simulink model "der"  (R2024b)
settings: Solver=VariableStepAuto  StartTime=0.0  StopTime=5  RelTol=1e-3
settings Model: Creator=32602  LastModifiedBy=32602

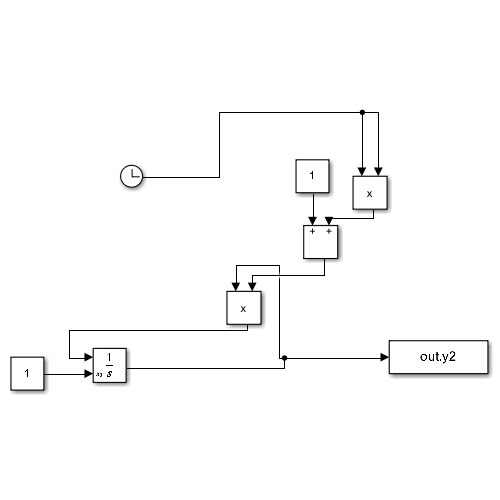
[thumbnail: Simulink's stored preview of the top-level diagram]
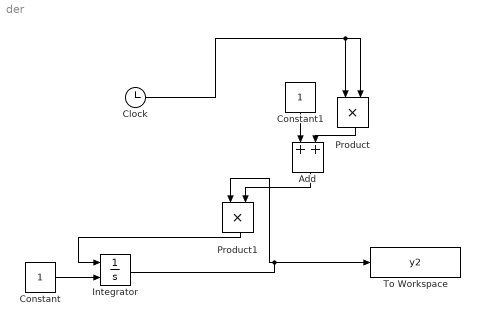
== system der ==
  Add : Sum
  Clock : Clock
  Constant : Constant
  Constant1 : Constant
  Integrator : Integrator  InitialConditionSource=external
  Product : Product
  Product1 : Product
  To Workspace : ToWorkspace  VariableName=y2  SaveFormat=Timeseries  SampleTime=0.01
  wires:
  Integrator/1 -> Product1/1, To Workspace/1
  Constant/1 -> Integrator/2
  Clock/1 -> Product/2, Product/1
  Constant1/1 -> Add/1
  Product/1 -> Add/2
  Add/1 -> Product1/2
  Product1/1 -> Integrator/1
